simulink model "campus_with_central_plant"  (Simulink 8.5)
settings: Solver=FixedStepDiscrete  StartTime=0.0  StopTime=Inf  FixedStep=300  RelTol=1e-3
undefined symbols (not defined in the file or in its folder): NREL, USA_CO_Golden
libraries: mlepLibrary x3
settings Model: Creator=wbernal  LastModifiedBy=wbernalh
settings DebuggingCC: SolverPrmCheckMsg=warning  FcnCallInpInsideContextMsg=EnableAllAsWarning

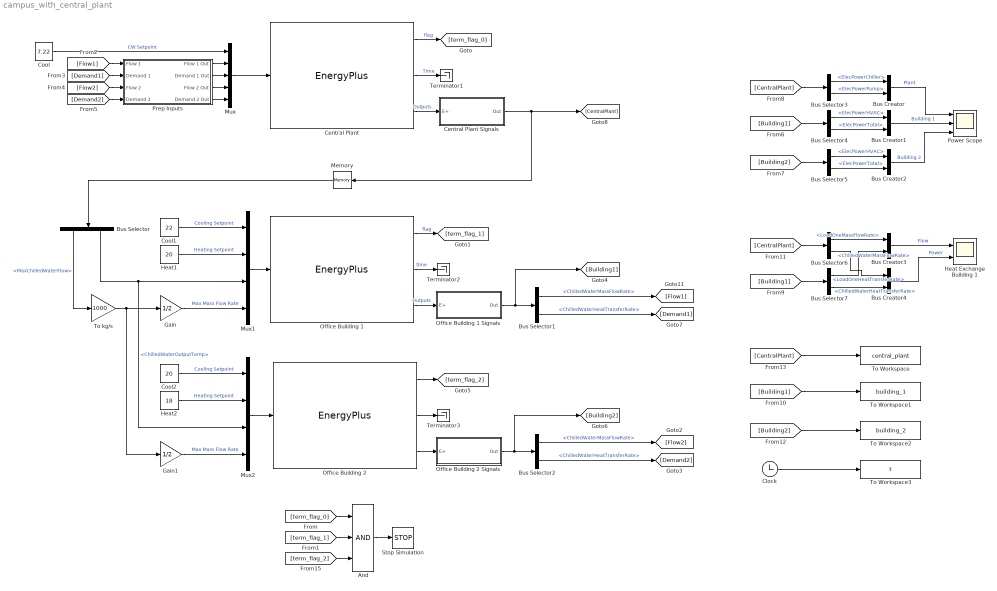
== system campus_with_central_plant ==
  And : Logic  Inputs=3  IconShape=distinctive  AllPortsSameDT=off  OutDataTypeStr=boolean
  Bus Creator{,1..4} (5 alike) : BusCreator  Inputs=2
  Bus Selector : BusSelector  OutputSignals=MaxChilledWaterFlow,ChilledWaterOutputTemp
  Bus Selector1 : BusSelector  OutputSignals=ChilledWaterMassFlowRate,ChilledWaterHeatTransferRate
  Bus Selector2 : BusSelector  OutputSignals=ChilledWaterMassFlowRate,ChilledWaterHeatTransferRate
  Bus Selector3 : BusSelector  OutputSignals=ElecPowerChiller,ElecPowerPump
  Bus Selector4 : BusSelector  OutputSignals=ElecPowerHVAC,ElecPowerTotal
  Bus Selector5 : BusSelector  OutputSignals=ElecPowerHVAC,ElecPowerTotal
  Bus Selector6 : BusSelector  OutputSignals=LoadOneMassFlowRate,LoadOneHeatTransferRate
  Bus Selector7 : BusSelector  OutputSignals=ChilledWaterMassFlowRate,ChilledWaterHeatTransferRate
  Central Plant : mlepLibrary/EnergyPlus  work_dir=ElectricChiller  rel_path=on  fname=ElectricChiller  weather_profile=USA_CO_Golden-NREL.724666_TMY3  time_step=300  nout=13  timeout=15  mlep_defaults=on  port=0
  Central Plant Signals : Subsystem
  Clock : Clock
  Cool : Constant  Value=7.22
  Cool1 : Constant  Value=22
  Cool2 : Constant  Value=20
  Gain : Gain  Gain=1/2
  Gain1 : Gain  Gain=1/2
  Heat Exchange Building 1 : Scope  NumInputPorts=2
      settings: ShowLegends=on  TimeRange=450000  YMin=0~-25000  YMax=5~0
  Heat1 : Constant  Value=20
  Heat2 : Constant  Value=18
  Memory : Memory
  Mux : Mux  Inputs=5
  Mux1 : Mux
  Mux2 : Mux
  Office Building 1 : mlepLibrary/EnergyPlus  work_dir=Building1  rel_path=on  fname=5ZoneAirCool  weather_profile=USA_CO_Golden-NREL.724666_TMY3  time_step=300  nout=13  timeout=15  mlep_defaults=on  port=0
  Office Building 1 Signals : Subsystem
  Office Building 2 : mlepLibrary/EnergyPlus  work_dir=Building2  rel_path=on  fname=5ZoneAirCool  weather_profile=USA_CO_Golden-NREL.724666_TMY3  time_step=300  nout=13  timeout=15  mlep_defaults=on  port=0
  Office Building 2 Signals : Subsystem
  Power Scope : Scope  NumInputPorts=3
      settings: ShowLegends=on  TimeRange=450000  YMin=0~0~0  YMax=10000~12000~12000
  Prep Inputs : Subsystem
  Stop Simulation : Stop
  Terminator1 : Terminator
  Terminator2 : Terminator
  Terminator3 : Terminator
  To Workspace : ToWorkspace  VariableName=central_plant  SampleTime=-1
  To Workspace1 : ToWorkspace  VariableName=building_1  SampleTime=-1
  To Workspace2 : ToWorkspace  VariableName=building_2  SampleTime=-1
  To Workspace3 : ToWorkspace  VariableName=t  SampleTime=-1
  To kg/s : Gain  Gain=1000
  wires:
  Cool/1 -> Mux/1  "CW Setpoint"
  Cool1/1 -> Mux1/1  "Cooling Setpoint"
  Heat1/1 -> Mux1/2  "Heating Setpoint"
  And/1 -> Stop Simulation/1
  [term_flag_0] -> And/1
  [term_flag_1] -> And/2
  Cool2/1 -> Mux2/1  "Cooling Setpoint"
  Heat2/1 -> Mux2/2  "Heating Setpoint"
  [term_flag_2] -> And/3
  Prep Inputs/1(Flow 1 Out) -> Mux/2
  Prep Inputs/2(Demand 1 Out) -> Mux/3
  Prep Inputs/3(Flow 2 Out) -> Mux/4
  Prep Inputs/4(Demand 2 Out) -> Mux/5
  Central Plant/1 -> [term_flag_0]  "flag"
  Office Building 1/1 -> [term_flag_1]  "flag"
  Central Plant/2 -> Terminator1/1  "Time"
  Office Building 1/2 -> Terminator2/1  "time"
  Office Building 2/2 -> Terminator3/1
  Office Building 2/1 -> [term_flag_2]
  Mux/1 -> Central Plant/1
  Central Plant/3 -> Central Plant Signals/1(E+)  "Outputs"
  Office Building 1/3 -> Office Building 1 Signals/1(E+)  "Outputs"
  Office Building 2/3 -> Office Building 2 Signals/1(E+)
  Central Plant Signals/1(Out) -> [CentralPlant], Memory/1
  Memory/1 -> Bus Selector/1
  Office Building 1 Signals/1(Out) -> [Building1], Bus Selector1/1
  Bus Selector1/2 -> [Demand1]  "<ChilledWaterHeatTransferRate>"
  Bus Selector1/1 -> [Flow1]  "<ChilledWaterMassFlowRate>"
  [Flow1] -> Prep Inputs/1(Flow 1)
  [Demand1] -> Prep Inputs/2(Demand 1)
  [Flow2] -> Prep Inputs/3(Flow 2)
  [Demand2] -> Prep Inputs/4(Demand 2)
  Mux1/1 -> Office Building 1/1
  Mux2/1 -> Office Building 2/1
  Bus Selector/2 -> Mux2/3, Mux1/3  "<ChilledWaterOutputTemp>"
  Bus Selector/1 -> To kg/s/1  "<MaxChilledWaterFlow>"
  To kg/s/1 -> Gain1/1, Gain/1
  Gain/1 -> Mux1/4  "Max Mass Flow Rate"
  Gain1/1 -> Mux2/4  "Max Mass Flow Rate"
  Bus Selector2/2 -> [Demand2]  "<ChilledWaterHeatTransferRate>"
  Bus Selector2/1 -> [Flow2]  "<ChilledWaterMassFlowRate>"
  Bus Selector3/1 -> Bus Creator/1  "<ElecPowerChiller>"
  Bus Selector3/2 -> Bus Creator/2  "<ElecPowerPump>"
  Bus Creator/1 -> Power Scope/1  "Plant"
  Bus Selector4/1 -> Bus Creator1/1  "<ElecPowerHVAC>"
  Bus Selector4/2 -> Bus Creator1/2  "<ElecPowerTotal>"
  Bus Selector5/1 -> Bus Creator2/1  "<ElecPowerHVAC>"
  Bus Selector5/2 -> Bus Creator2/2  "<ElecPowerTotal>"
  Bus Creator1/1 -> Power Scope/2  "Building 1"
  Bus Creator2/1 -> Power Scope/3  "Building 2"
  Office Building 2 Signals/1(Out) -> [Building2], Bus Selector2/1
  [CentralPlant] -> Bus Selector3/1
  [Building1] -> Bus Selector4/1
  [Building2] -> Bus Selector5/1
  [CentralPlant] -> Bus Selector6/1
  [Building1] -> Bus Selector7/1
  Bus Selector6/1 -> Bus Creator3/1  "<LoadOneMassFlowRate>"
  Bus Selector7/1 -> Bus Creator3/2  "<ChilledWaterMassFlowRate>"
  Bus Selector6/2 -> Bus Creator4/1  "<LoadOneHeatTransferRate>"
  Bus Selector7/2 -> Bus Creator4/2  "<ChilledWaterHeatTransferRate>"
  Bus Creator3/1 -> Heat Exchange Building 1/1  "Flow"
  Bus Creator4/1 -> Heat Exchange Building 1/2  "Power"
  [CentralPlant] -> To Workspace/1
  [Building1] -> To Workspace1/1
  [Building2] -> To Workspace2/1
  Clock/1 -> To Workspace3/1

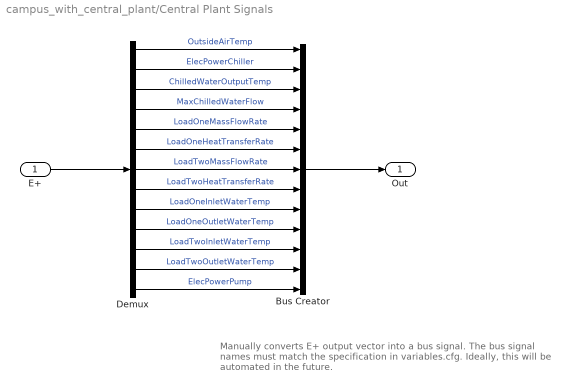
== system campus_with_central_plant/Central Plant Signals ==
  note: Manually converts E+ output vector into a bus signal.
      | The bus signal names must match the specification in variables.cfg.
      | Ideally, this will be automated in the future.
  E+ : Inport
  Bus Creator : BusCreator  Inputs=13
  Demux : Demux  Outputs=13
  Out : Outport
  wires:
  E+/1 -> Demux/1
  Bus Creator/1 -> Out/1
  Demux/1 -> Bus Creator/1  "OutsideAirTemp"
  Demux/2 -> Bus Creator/2  "ElecPowerChiller"
  Demux/3 -> Bus Creator/3  "ChilledWaterOutputTemp"
  Demux/4 -> Bus Creator/4  "MaxChilledWaterFlow"
  Demux/5 -> Bus Creator/5  "LoadOneMassFlowRate"
  Demux/6 -> Bus Creator/6  "LoadOneHeatTransferRate"
  Demux/7 -> Bus Creator/7  "LoadTwoMassFlowRate"
  Demux/8 -> Bus Creator/8  "LoadTwoHeatTransferRate"
  Demux/9 -> Bus Creator/9  "LoadOneInletWaterTemp"
  Demux/10 -> Bus Creator/10  "LoadOneOutletWaterTemp"
  Demux/11 -> Bus Creator/11  "LoadTwoInletWaterTemp"
  Demux/12 -> Bus Creator/12  "LoadTwoOutletWaterTemp"
  Demux/13 -> Bus Creator/13  "ElecPowerPump"

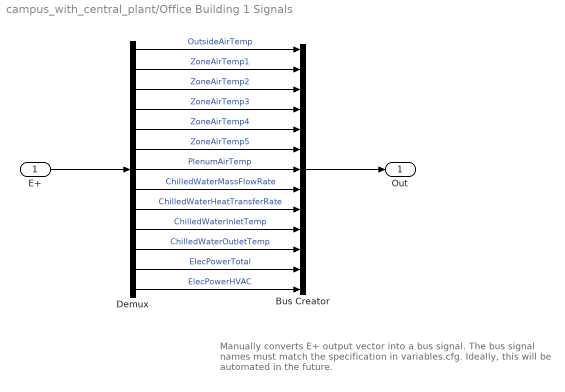
== system campus_with_central_plant/Office Building 1 Signals ==
  note: Manually converts E+ output vector into a bus signal.
      | The bus signal names must match the specification in variables.cfg.
      | Ideally, this will be automated in the future.
  E+ : Inport
  Bus Creator : BusCreator  Inputs=13
  Demux : Demux  Outputs=13
  Out : Outport
  wires:
  E+/1 -> Demux/1
  Bus Creator/1 -> Out/1
  Demux/1 -> Bus Creator/1  "OutsideAirTemp"
  Demux/2 -> Bus Creator/2  "ZoneAirTemp1"
  Demux/3 -> Bus Creator/3  "ZoneAirTemp2"
  Demux/4 -> Bus Creator/4  "ZoneAirTemp3"
  Demux/5 -> Bus Creator/5  "ZoneAirTemp4"
  Demux/6 -> Bus Creator/6  "ZoneAirTemp5"
  Demux/7 -> Bus Creator/7  "PlenumAirTemp"
  Demux/8 -> Bus Creator/8  "ChilledWaterMassFlowRate"
  Demux/9 -> Bus Creator/9  "ChilledWaterHeatTransferRate"
  Demux/10 -> Bus Creator/10  "ChilledWaterInletTemp"
  Demux/11 -> Bus Creator/11  "ChilledWaterOutletTemp"
  Demux/12 -> Bus Creator/12  "ElecPowerTotal"
  Demux/13 -> Bus Creator/13  "ElecPowerHVAC"

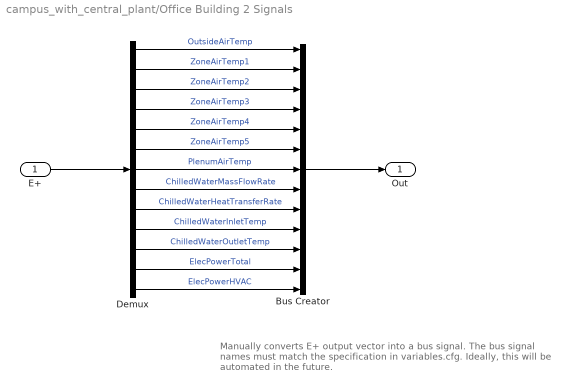
== system campus_with_central_plant/Office Building 2 Signals ==
  note: Manually converts E+ output vector into a bus signal.
      | The bus signal names must match the specification in variables.cfg.
      | Ideally, this will be automated in the future.
  E+ : Inport
  Bus Creator : BusCreator  Inputs=13
  Demux : Demux  Outputs=13
  Out : Outport
  wires:
  E+/1 -> Demux/1
  Bus Creator/1 -> Out/1
  Demux/1 -> Bus Creator/1  "OutsideAirTemp"
  Demux/2 -> Bus Creator/2  "ZoneAirTemp1"
  Demux/3 -> Bus Creator/3  "ZoneAirTemp2"
  Demux/4 -> Bus Creator/4  "ZoneAirTemp3"
  Demux/5 -> Bus Creator/5  "ZoneAirTemp4"
  Demux/6 -> Bus Creator/6  "ZoneAirTemp5"
  Demux/7 -> Bus Creator/7  "PlenumAirTemp"
  Demux/8 -> Bus Creator/8  "ChilledWaterMassFlowRate"
  Demux/9 -> Bus Creator/9  "ChilledWaterHeatTransferRate"
  Demux/10 -> Bus Creator/10  "ChilledWaterInletTemp"
  Demux/11 -> Bus Creator/11  "ChilledWaterOutletTemp"
  Demux/12 -> Bus Creator/12  "ElecPowerTotal"
  Demux/13 -> Bus Creator/13  "ElecPowerHVAC"

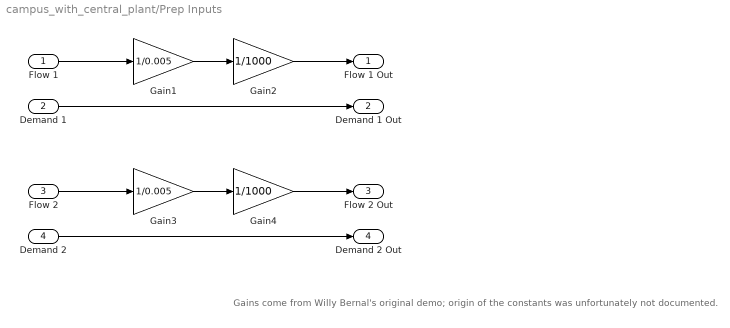
== system campus_with_central_plant/Prep Inputs ==
  note: Gains come from Willy Bernal's original demo; origin of the constants was unfortunately not documented.
  Flow 1 : Inport
  Demand 1 : Inport  Port=2
  Flow 2 : Inport  Port=3
  Demand 2 : Inport  Port=4
  Gain1 : Gain  Gain=1/0.005
  Gain2 : Gain  Gain=1/1000
  Gain3 : Gain  Gain=1/0.005
  Gain4 : Gain  Gain=1/1000
  Flow 1 Out : Outport
  Demand 1 Out : Outport  Port=2
  Flow 2 Out : Outport  Port=3
  Demand 2 Out : Outport  Port=4
  wires:
  Flow 1/1 -> Gain1/1
  Gain1/1 -> Gain2/1
  Gain2/1 -> Flow 1 Out/1
  Gain3/1 -> Gain4/1
  Demand 1/1 -> Demand 1 Out/1
  Flow 2/1 -> Gain3/1
  Gain4/1 -> Flow 2 Out/1
  Demand 2/1 -> Demand 2 Out/1
